simulink model "Modelos"  (R2025a)
settings: Solver=FixedStepDiscrete  StartTime=0.0  StopTime=P.Tsim  FixedStep=P.Ts  RelTol=1e-3
InitFcn:
  | CarregaDados
values from neighbouring files (symbols this model uses):
  P = struct    [CarregaDados.m]
(part 1 of 2)
settings Model: Creator=leize  LastModifiedBy=Rafael

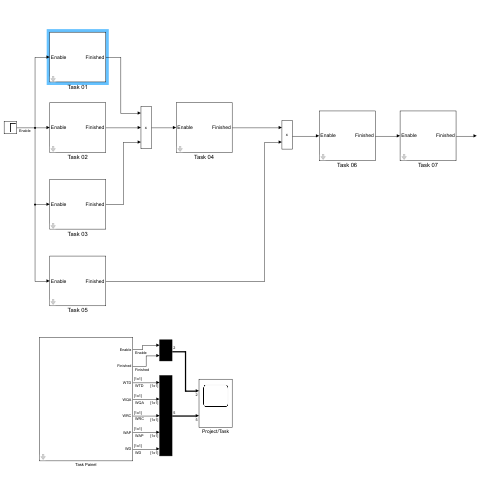
[thumbnail: Simulink's stored preview of the top-level diagram]
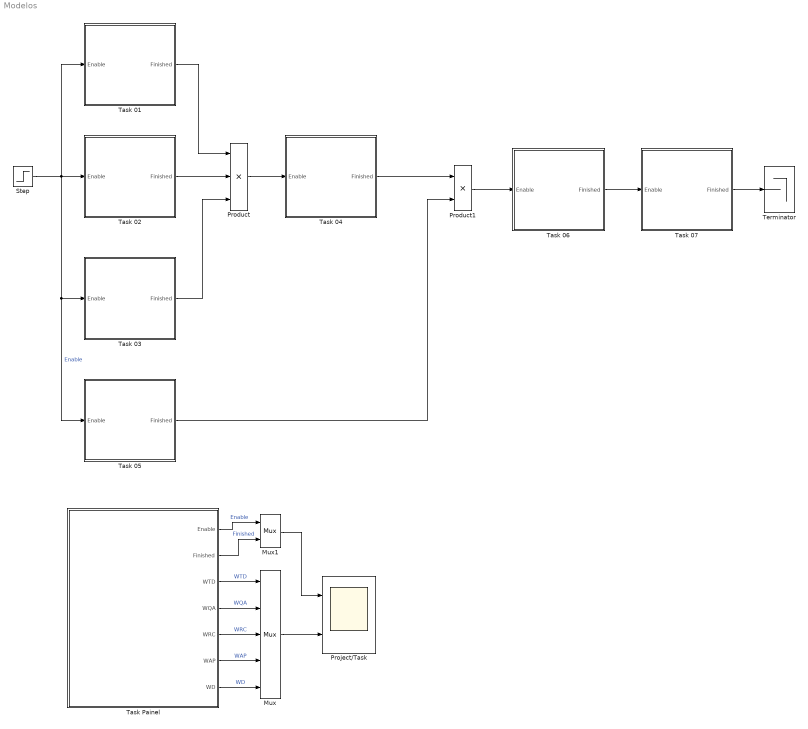
== system Modelos ==
  Mux : Mux  Inputs=5
  Mux1 : Mux  Inputs=2
  Product : Product  Inputs=3
  Product1 : Product
  Project/Task : Scope  NumInputPorts=2
      settings: ActiveDisplayYMinimum=-0.125  ActiveDisplayYMaximum=1.125  DataLoggingVariableName=ScopeData2
  Step : Step  Time=10  SampleTime=0
  Task 01 : Subsystem  mask{P=P, task_id=1}
      mask prompts: P "General task parameters"; task_id "Task Id (num)"
  Task 02 : Subsystem  mask{P=P, task_id=2}
      mask prompts: P "General task parameters"; task_id "Task Id (num)"
  Task 03 : Subsystem  mask{P=P, task_id=3}
      mask prompts: P "General task parameters"; task_id "Task Id (num)"
  Task 04 : Subsystem  mask{P=P, task_id=4}
      mask prompts: P "General task parameters"; task_id "Task Id (num)"
  Task 05 : Subsystem  mask{P=P, task_id=5}
      mask prompts: P "General task parameters"; task_id "Task Id (num)"
  Task 06 : Subsystem  mask{P=P, task_id=6}
      mask prompts: P "General task parameters"; task_id "Task Id (num)"
  Task 07 : Subsystem  mask{P=P, task_id=7}
      mask prompts: P "General task parameters"; task_id "Task Id (num)"
  Task Painel : Subsystem  mask{task_id=All Projet}
      mask prompts: task_id "Task Selecion"
  Terminator : Terminator
  wires:
  Task Painel/3(WTD) -> Mux/1  "WTD"
  Task Painel/6(WAP) -> Mux/4  "WAP"
  Task Painel/5(WRC) -> Mux/3  "WRC"
  Task Painel/4(WQA) -> Mux/2  "WQA"
  Task Painel/7(WD) -> Mux/5  "WD"
  Mux/1 -> Project/Task/2
  Step/1 -> Task 02/1(Enable), Task 01/1(Enable), Task 05/1(Enable), Task 03/1(Enable)  "Enable"
  Product/1 -> Task 04/1(Enable)
  Task 01/1(Finished) -> Product/1
  Task 02/1(Finished) -> Product/2
  Task 03/1(Finished) -> Product/3
  Task 04/1(Finished) -> Product1/1
  Task 05/1(Finished) -> Product1/2
  Product1/1 -> Task 06/1(Enable)
  Task 06/1(Finished) -> Task 07/1(Enable)
  Task 07/1(Finished) -> Terminator/1
  Mux1/1 -> Project/Task/1
  Task Painel/1(Enable) -> Mux1/1  "Enable"
  Task Painel/2(Finished) -> Mux1/2  "Finished"

== system Modelos/Task 01 ==
  Enable : Inport
  Controle : Subsystem
  Equações Modelo Discretizado : Subsystem
  MATLAB Function : MATLAB Function  TreatAsAtomicUnit=on
  Mux1 : Mux  Inputs=5
  Finished : Outport
  tag scope: Enable1=global, Finished1=global, W1=global
  wires:
  MATLAB Function/1(Done) -> Finished/1, [Finished1]  "Finished"
  Controle/1(Ações) -> Equações Modelo Discretizado/2(Ações)
  Enable/1 -> Equações Modelo Discretizado/1(Enable), MATLAB Function/1(enable), [Enable1]  "Enable"
  Equações Modelo Discretizado/3(Work Reviewing By Client) -> Mux1/3  "WRC"
  Equações Modelo Discretizado/1(Work To Do) -> Mux1/1  "WTD"
  Mux1/1 -> Controle/1(Estados Atuais), MATLAB Function/2(Work), [W1]
  Equações Modelo Discretizado/5(Work Done) -> Mux1/5  "WD"
  Equações Modelo Discretizado/4(Work Approved) -> Mux1/4  "WAP"
  Equações Modelo Discretizado/2("Work Awaiting quality assessment ") -> Mux1/2  "WQA"

== system Modelos/Task 02 ==
  Enable : Inport
  Controle : Subsystem
  Equações Modelo Discretizado : Subsystem
  MATLAB Function : MATLAB Function  TreatAsAtomicUnit=on
  Mux1 : Mux  Inputs=5
  Finished : Outport
  tag scope: Enable2=global, Finished2=global, W2=global
  wires:
  Equações Modelo Discretizado/2("Work Awaiting quality assessment ") -> Mux1/2  "WQA"
  Equações Modelo Discretizado/4(Work Approved) -> Mux1/4  "WAP"
  Equações Modelo Discretizado/5(Work Done) -> Mux1/5  "WD"
  Mux1/1 -> [W2], MATLAB Function/2(Work), Controle/1(Estados Atuais)
  Equações Modelo Discretizado/1(Work To Do) -> Mux1/1  "WTD"
  Equações Modelo Discretizado/3(Work Reviewing By Client) -> Mux1/3  "WRC"
  Enable/1 -> [Enable2], MATLAB Function/1(enable), Equações Modelo Discretizado/1(Enable)  "Enable"
  Controle/1(Ações) -> Equações Modelo Discretizado/2(Ações)
  MATLAB Function/1(Done) -> [Finished2], Finished/1  "Finished"

== system Modelos/Task 03 ==
  Enable : Inport
  Controle : Subsystem
  Equações Modelo Discretizado : Subsystem
  MATLAB Function : MATLAB Function  TreatAsAtomicUnit=on
  Mux1 : Mux  Inputs=5
  Finished : Outport
  tag scope: Enable3=global, Finished3=global, W3=global
  wires:
  MATLAB Function/1(Done) -> Finished/1, [Finished3]  "Finished"
  Controle/1(Ações) -> Equações Modelo Discretizado/2(Ações)
  Enable/1 -> Equações Modelo Discretizado/1(Enable), MATLAB Function/1(enable), [Enable3]  "Enable"
  Equações Modelo Discretizado/3(Work Reviewing By Client) -> Mux1/3  "WRC"
  Equações Modelo Discretizado/1(Work To Do) -> Mux1/1  "WTD"
  Mux1/1 -> Controle/1(Estados Atuais), MATLAB Function/2(Work), [W3]
  Equações Modelo Discretizado/5(Work Done) -> Mux1/5  "WD"
  Equações Modelo Discretizado/4(Work Approved) -> Mux1/4  "WAP"
  Equações Modelo Discretizado/2("Work Awaiting quality assessment ") -> Mux1/2  "WQA"

== system Modelos/Task 04 ==
  Enable : Inport
  Controle : Subsystem
  Equações Modelo Discretizado : Subsystem
  MATLAB Function : MATLAB Function  TreatAsAtomicUnit=on
  Mux1 : Mux  Inputs=5
  Finished : Outport
  tag scope: Enable4=global, Finished4=global, W4=global
  wires:
  Equações Modelo Discretizado/2("Work Awaiting quality assessment ") -> Mux1/2  "WQA"
  Equações Modelo Discretizado/4(Work Approved) -> Mux1/4  "WAP"
  Equações Modelo Discretizado/5(Work Done) -> Mux1/5  "WD"
  Mux1/1 -> [W4], MATLAB Function/2(Work), Controle/1(Estados Atuais)
  Equações Modelo Discretizado/1(Work To Do) -> Mux1/1  "WTD"
  Equações Modelo Discretizado/3(Work Reviewing By Client) -> Mux1/3  "WRC"
  Enable/1 -> [Enable4], MATLAB Function/1(enable), Equações Modelo Discretizado/1(Enable)  "Enable"
  Controle/1(Ações) -> Equações Modelo Discretizado/2(Ações)
  MATLAB Function/1(Done) -> [Finished4], Finished/1  "Finished"

== system Modelos/Task 05 ==
  Enable : Inport
  Controle : Subsystem
  Equações Modelo Discretizado : Subsystem
  MATLAB Function : MATLAB Function  TreatAsAtomicUnit=on
  Mux1 : Mux  Inputs=5
  Finished : Outport
  tag scope: Enable5=global, Finished5=global, W5=global
  wires:
  MATLAB Function/1(Done) -> Finished/1, [Finished5]  "Finished"
  Controle/1(Ações) -> Equações Modelo Discretizado/2(Ações)
  Enable/1 -> Equações Modelo Discretizado/1(Enable), MATLAB Function/1(enable), [Enable5]  "Enable"
  Equações Modelo Discretizado/3(Work Reviewing By Client) -> Mux1/3  "WRC"
  Equações Modelo Discretizado/1(Work To Do) -> Mux1/1  "WTD"
  Mux1/1 -> Controle/1(Estados Atuais), MATLAB Function/2(Work), [W5]
  Equações Modelo Discretizado/5(Work Done) -> Mux1/5  "WD"
  Equações Modelo Discretizado/4(Work Approved) -> Mux1/4  "WAP"
  Equações Modelo Discretizado/2("Work Awaiting quality assessment ") -> Mux1/2  "WQA"

== system Modelos/Task 06 ==
  Enable : Inport
  Controle : Subsystem
  Equações Modelo Discretizado : Subsystem
  MATLAB Function : MATLAB Function  TreatAsAtomicUnit=on
  Mux1 : Mux  Inputs=5
  Finished : Outport
  tag scope: Enable6=global, Finished6=global, W6=global
  wires:
  MATLAB Function/1(Done) -> Finished/1, [Finished6]  "Finished"
  Controle/1(Ações) -> Equações Modelo Discretizado/2(Ações)
  Enable/1 -> Equações Modelo Discretizado/1(Enable), MATLAB Function/1(enable), [Enable6]  "Enable"
  Equações Modelo Discretizado/3(Work Reviewing By Client) -> Mux1/3  "WRC"
  Equações Modelo Discretizado/1(Work To Do) -> Mux1/1  "WTD"
  Mux1/1 -> Controle/1(Estados Atuais), MATLAB Function/2(Work), [W6]
  Equações Modelo Discretizado/5(Work Done) -> Mux1/5  "WD"
  Equações Modelo Discretizado/4(Work Approved) -> Mux1/4  "WAP"
  Equações Modelo Discretizado/2("Work Awaiting quality assessment ") -> Mux1/2  "WQA"

== system Modelos/Task 07 ==
  Enable : Inport
  Controle : Subsystem
  Equações Modelo Discretizado : Subsystem
  MATLAB Function : MATLAB Function  TreatAsAtomicUnit=on
  Mux1 : Mux  Inputs=5
  Finished : Outport
  tag scope: Enable7=global, Finished7=global, W7=global
  wires:
  Equações Modelo Discretizado/2("Work Awaiting quality assessment ") -> Mux1/2  "WQA"
  Equações Modelo Discretizado/4(Work Approved) -> Mux1/4  "WAP"
  Equações Modelo Discretizado/5(Work Done) -> Mux1/5  "WD"
  Mux1/1 -> [W7], MATLAB Function/2(Work), Controle/1(Estados Atuais)
  Equações Modelo Discretizado/1(Work To Do) -> Mux1/1  "WTD"
  Equações Modelo Discretizado/3(Work Reviewing By Client) -> Mux1/3  "WRC"
  Enable/1 -> [Enable7], MATLAB Function/1(enable), Equações Modelo Discretizado/1(Enable)  "Enable"
  Controle/1(Ações) -> Equações Modelo Discretizado/2(Ações)
  MATLAB Function/1(Done) -> [Finished7], Finished/1  "Finished"

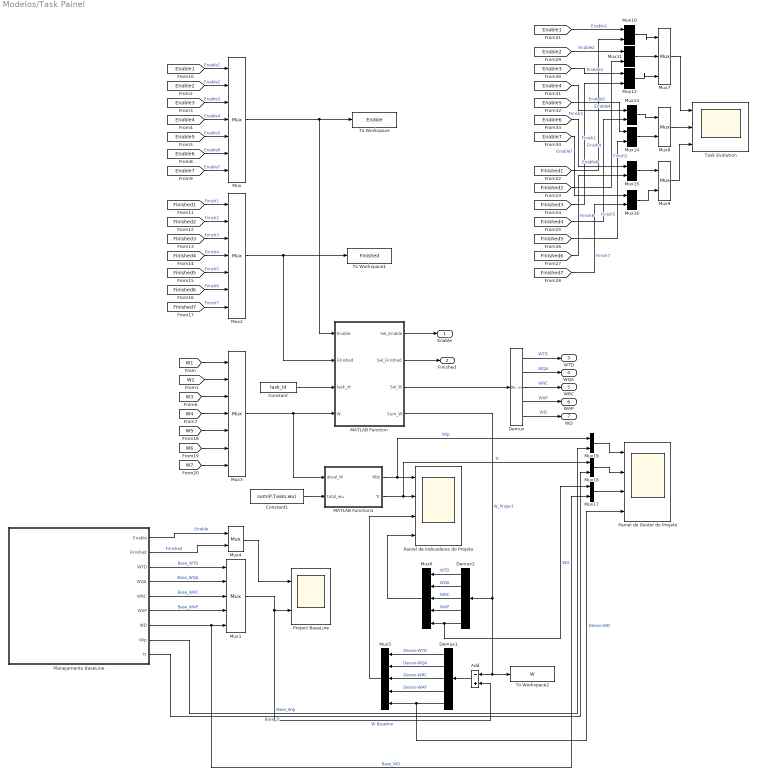
== system Modelos/Task Painel ==
  Add : Sum  Inputs=-+
  Constant : Constant  Value=task_id
  Constant1 : Constant  Value=sum(P.Tasks.wu)
  Demux : Demux  Outputs=5
  Demux1 : Demux  Outputs=5
  Demux2 : Demux  Outputs=5
  MATLAB Function : MATLAB Function  TreatAsAtomicUnit=on
  MATLAB Function1 : MATLAB Function  TreatAsAtomicUnit=on
  Mux : Mux  Inputs=7
  Mux1 : Mux  Inputs=5
  Mux{4,8..19} (13 alike) : Mux  Inputs=2
  Mux2 : Mux  Inputs=7
  Mux3 : Mux  Inputs=7
  Mux5 : Mux  Inputs=5
  Mux6 : Mux  Inputs=5
  Mux7 : Mux  Inputs=3
  Painel de Indicadores do Projeto : Scope  NumInputPorts=4
      settings: ActiveDisplayYMinimum=-25806.89231  ActiveDisplayYMaximum=232262.03078
  Painel do Gestor do Projeto : Scope  NumInputPorts=4
      settings: ActiveDisplayYMinimum=-25804.64462  ActiveDisplayYMaximum=232241.80155  DataLoggingVariableName=ScopeData2
  Planejamento BaseLine : Subsystem
  Project BaseLine : Scope  NumInputPorts=2
      settings: ActiveDisplayYMinimum=-0.125  ActiveDisplayYMaximum=1.125  DataLoggingVariableName=ScopeData2
  Task Evolution : Scope  NumInputPorts=3
      settings: ActiveDisplayYMinimum=-0.125  ActiveDisplayYMaximum=1.125
  To Workspace : ToWorkspace  VariableName=Enable  SampleTime=P.Ts
      settings: Save2DSignal=2-D array (concatenate along first dimension)
  To Workspace1 : ToWorkspace  VariableName=Finished  SampleTime=P.Ts
      settings: Save2DSignal=2-D array (concatenate along first dimension)
  To Workspace2 : ToWorkspace  VariableName=W  SampleTime=P.Ts
      settings: Save2DSignal=2-D array (concatenate along first dimension)
  Enable : Outport
  Finished : Outport  Port=2
  WTD : Outport  Port=3
  WQA : Outport  Port=4
  WRC : Outport  Port=5
  WAP : Outport  Port=6
  WD : Outport  Port=7
  wires:
  [W1] -> Mux3/1
  [W2] -> Mux3/2
  Demux/1 -> WTD/1  "WTD"
  Demux/2 -> WQA/1  "WQA"
  Demux/3 -> WRC/1  "WRC"
  Demux/4 -> WAP/1  "WAP"
  Demux/5 -> WD/1  "WD"
  Constant/1 -> MATLAB Function/3(task_id)
  [Enable2] -> Mux/2  "Enable2"
  [Enable3] -> Mux/3  "Enable3"
  Mux/1 -> To Workspace/1, MATLAB Function/1(Enable)
  [Enable4] -> Mux/4  "Enable4"
  [Enable5] -> Mux/5  "Enable5"
  [W3] -> Mux3/3
  [W4] -> Mux3/4
  [Enable6] -> Mux/6  "Enable6"
  [Enable7] -> Mux/7  "Enable7"
  [Enable1] -> Mux/1  "Enable1"
  [Finished1] -> Mux2/1  "Finish1"
  [Finished7] -> Mux2/7  "Finish7"
  [Finished6] -> Mux2/6  "Finish6"
  [Finished5] -> Mux2/5  "Finish5"
  [Finished4] -> Mux2/4  "Finish4"
  Mux2/1 -> To Workspace1/1, MATLAB Function/2(Finished)
  [Finished3] -> Mux2/3  "Finish3"
  [Finished2] -> Mux2/2  "Finish2"
  [W5] -> Mux3/5
  [W6] -> Mux3/6
  [W7] -> Mux3/7
  Mux3/1 -> MATLAB Function1/1(atual_W), MATLAB Function/4(W)
  MATLAB Function/1(Sel_Enable) -> Enable/1
  MATLAB Function/2(Sel_Finished) -> Finished/1
  Constant1/1 -> MATLAB Function1/2(total_wu)
  MATLAB Function1/1(Wip) -> Mux19/1, Painel de Indicadores do Projeto/1  "Wip"
  MATLAB Function1/2(Tr) -> Mux18/1, Painel de Indicadores do Projeto/2  "Tr"
  Planejamento BaseLine/1(Enable) -> Mux4/1  "Enable"
  Planejamento BaseLine/5(WRC) -> Mux1/3  "Base_WRC"
  Planejamento BaseLine/6(WAP) -> Mux1/4  "Base_WAP"
  Planejamento BaseLine/7(WD) -> Mux17/2, Mux1/5  "Base_WD"
  Planejamento BaseLine/3(WTD) -> Mux1/1  "Base_WTD"
  Mux4/1 -> Project BaseLine/1
  Mux1/1 -> Add/2, Project BaseLine/2  "W Baseline"
  Planejamento BaseLine/4(WQA) -> Mux1/2  "Base_WQA"
  MATLAB Function/3(Sel_W) -> Demux/1
  Planejamento BaseLine/2(Finished) -> Mux4/2  "Finished"
  MATLAB Function/4(Sum_W) -> Demux2/1, To Workspace2/1, Add/1  "W_Project"
  Add/1 -> Demux1/1
  Demux1/1 -> Mux5/1  "Desvio-WTD"
  Demux1/2 -> Mux5/2  "Desvio-WQA"
  Demux1/3 -> Mux5/3  "Desvio-WRC"
  Demux1/4 -> Mux5/4  "Desvio-WAP"
  Demux1/5 -> Painel do Gestor do Projeto/4, Mux5/5  "Desvio-WD"
  Mux5/1 -> Painel de Indicadores do Projeto/3
  Mux6/1 -> Painel de Indicadores do Projeto/4
  Demux2/5 -> Mux17/1, Mux6/5  "WD"
  Demux2/4 -> Mux6/4  "WAP"
  Demux2/3 -> Mux6/3  "WRC"
  Demux2/2 -> Mux6/2  "WQA"
  Demux2/1 -> Mux6/1  "WTD"
  [Enable4] -> Mux13/1  "Enable4"
  [Finished7] -> Mux16/2  "Finish7"
  [Enable3] -> Mux12/1  "Enable3"
  [Enable5] -> Mux14/1  "Enable5"
  [Finished1] -> Mux10/2  "Finish1"
  [Finished3] -> Mux12/2  "Finish3"
  [Finished5] -> Mux14/2  "Finish5"
  [Enable1] -> Mux10/1  "Enable1"
  [Finished4] -> Mux13/2  "Finish4"
  [Finished2] -> Mux11/2  "Finish2"
  [Finished6] -> Mux15/2  "Finish6"
  [Enable2] -> Mux11/1  "Enable2"
  [Enable6] -> Mux15/1  "Enable6"
  [Enable7] -> Mux16/1  "Enable7"
  Mux12/1 -> Mux7/3
  Mux11/1 -> Mux7/2
  Mux10/1 -> Mux7/1
  Mux7/1 -> Task Evolution/1
  Mux8/1 -> Task Evolution/2
  Mux9/1 -> Task Evolution/3
  Mux13/1 -> Mux8/1
  Mux14/1 -> Mux8/2
  Mux15/1 -> Mux9/1
  Mux16/1 -> Mux9/2
  Mux17/1 -> Painel do Gestor do Projeto/3
  Mux18/1 -> Painel do Gestor do Projeto/2
  Mux19/1 -> Painel do Gestor do Projeto/1
  Planejamento BaseLine/8(Wip) -> Mux19/2  "Base_Wip"
  Planejamento BaseLine/9(Tr) -> Mux18/2  "Base_Tr"

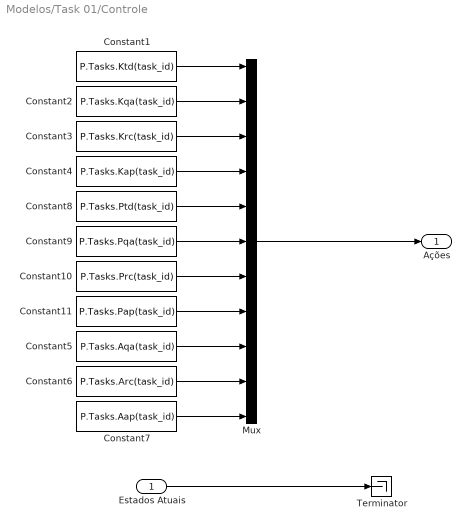
== system Modelos/Task 01/Controle ==
  Estados Atuais : Inport
  Constant1 : Constant  Value=P.Tasks.Ktd(task_id)
  Constant10 : Constant  Value=P.Tasks.Prc(task_id)
  Constant11 : Constant  Value=P.Tasks.Pap(task_id)
  Constant2 : Constant  Value=P.Tasks.Kqa(task_id)
  Constant3 : Constant  Value=P.Tasks.Krc(task_id)
  Constant4 : Constant  Value=P.Tasks.Kap(task_id)
  Constant5 : Constant  Value=P.Tasks.Aqa(task_id)
  Constant6 : Constant  Value=P.Tasks.Arc(task_id)
  Constant7 : Constant  Value=P.Tasks.Aap(task_id)
  Constant8 : Constant  Value=P.Tasks.Ptd(task_id)
  Constant9 : Constant  Value=P.Tasks.Pqa(task_id)
  Mux : Mux  Inputs=11
  Terminator : Terminator
  Ações : Outport
  wires:
  Estados Atuais/1 -> Terminator/1
  Constant1/1 -> Mux/1
  Constant4/1 -> Mux/4
  Constant3/1 -> Mux/3
  Constant2/1 -> Mux/2
  Mux/1 -> Ações/1
  Constant5/1 -> Mux/9
  Constant6/1 -> Mux/10
  Constant7/1 -> Mux/11
  Constant10/1 -> Mux/7
  Constant11/1 -> Mux/8
  Constant9/1 -> Mux/6
  Constant8/1 -> Mux/5

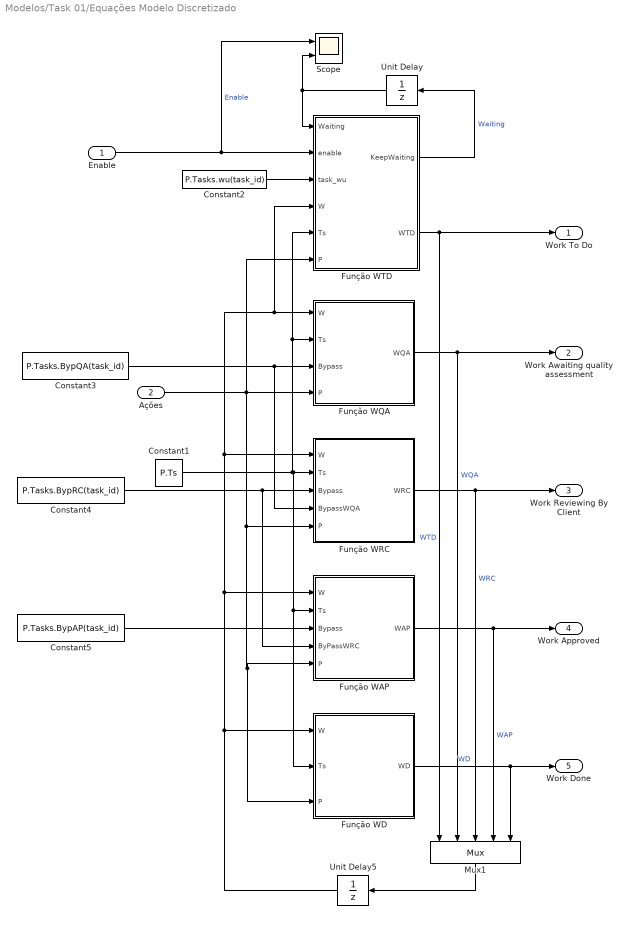
== system Modelos/Task 01/Equações Modelo Discretizado ==
  Enable : Inport
  Ações : Inport  Port=2
  Constant1 : Constant  Value=P.Ts  SampleTime=1
  Constant2 : Constant  Value=P.Tasks.wu(task_id)
  Constant3 : Constant  Value=P.Tasks.BypQA(task_id)  SampleTime=1
  Constant4 : Constant  Value=P.Tasks.BypRC(task_id)  SampleTime=1
  Constant5 : Constant  Value=P.Tasks.BypAP(task_id)  SampleTime=1
  Função WAP : MATLAB Function  TreatAsAtomicUnit=on
  Função WD : MATLAB Function  TreatAsAtomicUnit=on
  Função WQA : MATLAB Function  TreatAsAtomicUnit=on
  Função WRC : MATLAB Function  TreatAsAtomicUnit=on
  Função WTD : MATLAB Function  TreatAsAtomicUnit=on
  Mux1 : Mux  Inputs=5
  Scope : Scope  NumInputPorts=2
      settings: ActiveDisplayYMinimum=-0.125  ActiveDisplayYMaximum=1.125  DataLoggingVariableName=ScopeData2
  Unit Delay : UnitDelay  InitialCondition=1  SampleTime=-1  HasFrameUpgradeWarning=on
  Unit Delay5 : UnitDelay  InitialCondition=[P.Tasks.WTDini(task_id); P.Tasks.WQAini(task_id); P.Tasks.WRCini(task_id); P.Tasks.WAPini(task_id); P.Tasks.WDini(task_id)]  SampleTime=-1  HasFrameUpgradeWarning=on
  Work To Do : Outport
  "Work Awaiting quality assessment " : Outport  Port=2
  Work Reviewing By Client : Outport  Port=3
  Work Approved : Outport  Port=4
  Work Done : Outport  Port=5
  wires:
  Constant2/1 -> Função WTD/3(task_wu)
  Unit Delay/1 -> Scope/2, Função WTD/1(Waiting)
  Função WTD/1(KeepWaiting) -> Unit Delay/1  "Waiting"
  Função WD/1(WD) -> Mux1/5, Work Done/1  "WD"
  Constant1/1 -> Função WD/2(Ts), Função WAP/2(Ts), Função WRC/2(Ts), Função WQA/2(Ts), Função WTD/5(Ts)
  Unit Delay5/1 -> Função WD/1(W), Função WQA/1(W), Função WTD/4(W), Função WRC/1(W), Função WAP/1(W)
  Ações/1 -> Função WTD/6(P), Função WAP/5(P), Função WD/3(P), Função WRC/5(P), Função WQA/4(P)
  Mux1/1 -> Unit Delay5/1
  Enable/1 -> Função WTD/2(enable), Scope/1  "Enable"
  Função WAP/1(WAP) -> Mux1/4, Work Approved/1  "WAP"
  Função WRC/1(WRC) -> Mux1/3, Work Reviewing By Client/1  "WRC"
  Função WTD/2(WTD) -> Mux1/1, Work To Do/1  "WTD"
  Função WQA/1(WQA) -> Mux1/2, "Work Awaiting quality assessment "/1  "WQA"
  Constant3/1 -> Função WRC/4(BypassWQA), Função WQA/3(Bypass)
  Constant4/1 -> Função WAP/4(ByPassWRC), Função WRC/3(Bypass)
  Constant5/1 -> Função WAP/3(Bypass)

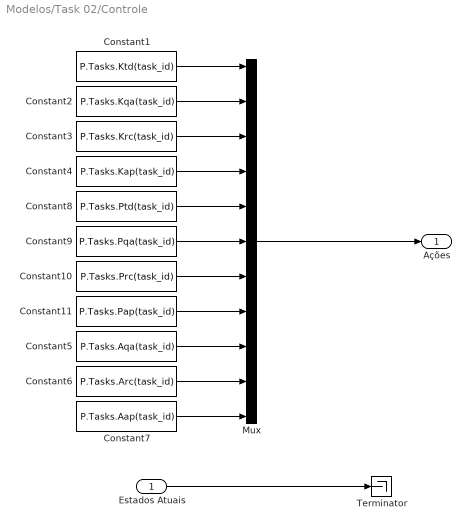
== system Modelos/Task 02/Controle ==
  Estados Atuais : Inport
  Constant1 : Constant  Value=P.Tasks.Ktd(task_id)
  Constant10 : Constant  Value=P.Tasks.Prc(task_id)
  Constant11 : Constant  Value=P.Tasks.Pap(task_id)
  Constant2 : Constant  Value=P.Tasks.Kqa(task_id)
  Constant3 : Constant  Value=P.Tasks.Krc(task_id)
  Constant4 : Constant  Value=P.Tasks.Kap(task_id)
  Constant5 : Constant  Value=P.Tasks.Aqa(task_id)
  Constant6 : Constant  Value=P.Tasks.Arc(task_id)
  Constant7 : Constant  Value=P.Tasks.Aap(task_id)
  Constant8 : Constant  Value=P.Tasks.Ptd(task_id)
  Constant9 : Constant  Value=P.Tasks.Pqa(task_id)
  Mux : Mux  Inputs=11
  Terminator : Terminator
  Ações : Outport
  wires:
  Constant8/1 -> Mux/5
  Constant9/1 -> Mux/6
  Constant11/1 -> Mux/8
  Constant10/1 -> Mux/7
  Constant7/1 -> Mux/11
  Constant6/1 -> Mux/10
  Constant5/1 -> Mux/9
  Mux/1 -> Ações/1
  Constant2/1 -> Mux/2
  Constant3/1 -> Mux/3
  Constant4/1 -> Mux/4
  Constant1/1 -> Mux/1
  Estados Atuais/1 -> Terminator/1

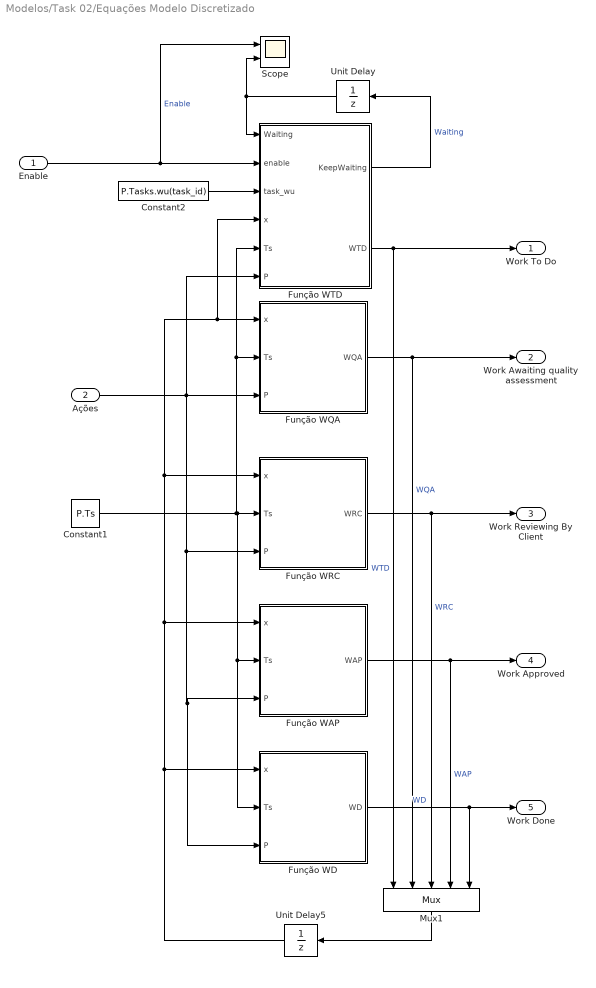
== system Modelos/Task 02/Equações Modelo Discretizado ==
  Enable : Inport
  Ações : Inport  Port=2
  Constant1 : Constant  Value=P.Ts  SampleTime=1
  Constant2 : Constant  Value=P.Tasks.wu(task_id)
  Função WAP : MATLAB Function  TreatAsAtomicUnit=on
  Função WD : MATLAB Function  TreatAsAtomicUnit=on
  Função WQA : MATLAB Function  TreatAsAtomicUnit=on
  Função WRC : MATLAB Function  TreatAsAtomicUnit=on
  Função WTD : MATLAB Function  TreatAsAtomicUnit=on
  Mux1 : Mux  Inputs=5
  Scope : Scope  NumInputPorts=2
      settings: ActiveDisplayYMinimum=-0.125  ActiveDisplayYMaximum=1.125  DataLoggingVariableName=ScopeData2
  Unit Delay : UnitDelay  InitialCondition=1  SampleTime=-1  HasFrameUpgradeWarning=on
  Unit Delay5 : UnitDelay  InitialCondition=[P.Tasks.WTDini(task_id); P.Tasks.WQAini(task_id); P.Tasks.WRCini(task_id); P.Tasks.WAPini(task_id); P.Tasks.WDini(task_id)]  SampleTime=-1  HasFrameUpgradeWarning=on
  Work To Do : Outport
  "Work Awaiting quality assessment " : Outport  Port=2
  Work Reviewing By Client : Outport  Port=3
  Work Approved : Outport  Port=4
  Work Done : Outport  Port=5
  wires:
  Função WQA/1(WQA) -> "Work Awaiting quality assessment "/1, Mux1/2  "WQA"
  Função WTD/2(WTD) -> Work To Do/1, Mux1/1  "WTD"
  Função WRC/1(WRC) -> Work Reviewing By Client/1, Mux1/3  "WRC"
  Função WAP/1(WAP) -> Work Approved/1, Mux1/4  "WAP"
  Enable/1 -> Scope/1, Função WTD/2(enable)  "Enable"
  Mux1/1 -> Unit Delay5/1
  Ações/1 -> Função WD/3(P), Função WAP/3(P), Função WRC/3(P), Função WTD/6(P), Função WQA/3(P)
  Unit Delay5/1 -> Função WRC/1(x), Função WTD/4(x), Função WQA/1(x), Função WAP/1(x), Função WD/1(x)
  Constant1/1 -> Função WRC/2(Ts), Função WD/2(Ts), Função WAP/2(Ts), Função WTD/5(Ts), Função WQA/2(Ts)
  Função WD/1(WD) -> Work Done/1, Mux1/5  "WD"
  Função WTD/1(KeepWaiting) -> Unit Delay/1  "Waiting"
  Unit Delay/1 -> Função WTD/1(Waiting), Scope/2
  Constant2/1 -> Função WTD/3(task_wu)

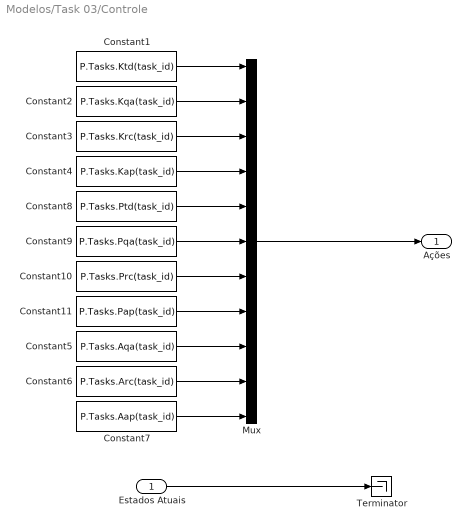
== system Modelos/Task 03/Controle ==
  Estados Atuais : Inport
  Constant1 : Constant  Value=P.Tasks.Ktd(task_id)
  Constant10 : Constant  Value=P.Tasks.Prc(task_id)
  Constant11 : Constant  Value=P.Tasks.Pap(task_id)
  Constant2 : Constant  Value=P.Tasks.Kqa(task_id)
  Constant3 : Constant  Value=P.Tasks.Krc(task_id)
  Constant4 : Constant  Value=P.Tasks.Kap(task_id)
  Constant5 : Constant  Value=P.Tasks.Aqa(task_id)
  Constant6 : Constant  Value=P.Tasks.Arc(task_id)
  Constant7 : Constant  Value=P.Tasks.Aap(task_id)
  Constant8 : Constant  Value=P.Tasks.Ptd(task_id)
  Constant9 : Constant  Value=P.Tasks.Pqa(task_id)
  Mux : Mux  Inputs=11
  Terminator : Terminator
  Ações : Outport
  wires:
  Estados Atuais/1 -> Terminator/1
  Constant1/1 -> Mux/1
  Constant4/1 -> Mux/4
  Constant3/1 -> Mux/3
  Constant2/1 -> Mux/2
  Mux/1 -> Ações/1
  Constant5/1 -> Mux/9
  Constant6/1 -> Mux/10
  Constant7/1 -> Mux/11
  Constant10/1 -> Mux/7
  Constant11/1 -> Mux/8
  Constant9/1 -> Mux/6
  Constant8/1 -> Mux/5

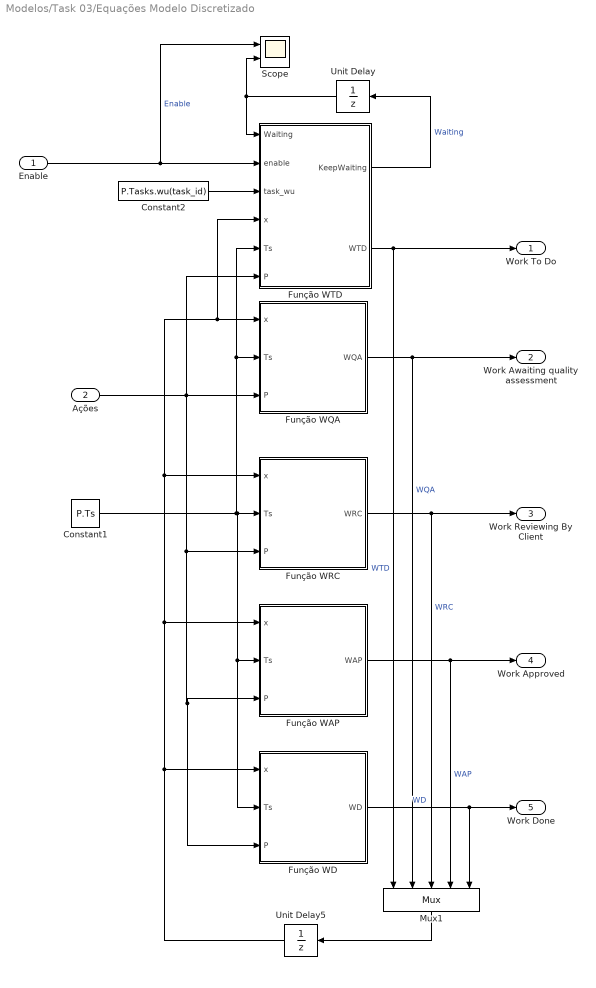
== system Modelos/Task 03/Equações Modelo Discretizado ==
  Enable : Inport
  Ações : Inport  Port=2
  Constant1 : Constant  Value=P.Ts  SampleTime=1
  Constant2 : Constant  Value=P.Tasks.wu(task_id)
  Função WAP : MATLAB Function  TreatAsAtomicUnit=on
  Função WD : MATLAB Function  TreatAsAtomicUnit=on
  Função WQA : MATLAB Function  TreatAsAtomicUnit=on
  Função WRC : MATLAB Function  TreatAsAtomicUnit=on
  Função WTD : MATLAB Function  TreatAsAtomicUnit=on
  Mux1 : Mux  Inputs=5
  Scope : Scope  NumInputPorts=2
      settings: ActiveDisplayYMinimum=-0.125  ActiveDisplayYMaximum=1.125  DataLoggingVariableName=ScopeData2
  Unit Delay : UnitDelay  InitialCondition=1  SampleTime=-1  HasFrameUpgradeWarning=on
  Unit Delay5 : UnitDelay  InitialCondition=[P.Tasks.WTDini(task_id); P.Tasks.WQAini(task_id); P.Tasks.WRCini(task_id); P.Tasks.WAPini(task_id); P.Tasks.WDini(task_id)]  SampleTime=-1  HasFrameUpgradeWarning=on
  Work To Do : Outport
  "Work Awaiting quality assessment " : Outport  Port=2
  Work Reviewing By Client : Outport  Port=3
  Work Approved : Outport  Port=4
  Work Done : Outport  Port=5
  wires:
  Constant2/1 -> Função WTD/3(task_wu)
  Unit Delay/1 -> Scope/2, Função WTD/1(Waiting)
  Função WTD/1(KeepWaiting) -> Unit Delay/1  "Waiting"
  Função WD/1(WD) -> Mux1/5, Work Done/1  "WD"
  Constant1/1 -> Função WQA/2(Ts), Função WTD/5(Ts), Função WAP/2(Ts), Função WD/2(Ts), Função WRC/2(Ts)
  Unit Delay5/1 -> Função WD/1(x), Função WAP/1(x), Função WQA/1(x), Função WTD/4(x), Função WRC/1(x)
  Ações/1 -> Função WQA/3(P), Função WTD/6(P), Função WRC/3(P), Função WAP/3(P), Função WD/3(P)
  Mux1/1 -> Unit Delay5/1
  Enable/1 -> Função WTD/2(enable), Scope/1  "Enable"
  Função WAP/1(WAP) -> Mux1/4, Work Approved/1  "WAP"
  Função WRC/1(WRC) -> Mux1/3, Work Reviewing By Client/1  "WRC"
  Função WTD/2(WTD) -> Mux1/1, Work To Do/1  "WTD"
  Função WQA/1(WQA) -> Mux1/2, "Work Awaiting quality assessment "/1  "WQA"

== system Modelos/Task 04/Controle ==
  Estados Atuais : Inport
  Constant1 : Constant  Value=P.Tasks.Ktd(task_id)
  Constant10 : Constant  Value=P.Tasks.Prc(task_id)
  Constant11 : Constant  Value=P.Tasks.Pap(task_id)
  Constant2 : Constant  Value=P.Tasks.Kqa(task_id)
  Constant3 : Constant  Value=P.Tasks.Krc(task_id)
  Constant4 : Constant  Value=P.Tasks.Kap(task_id)
  Constant5 : Constant  Value=P.Tasks.Aqa(task_id)
  Constant6 : Constant  Value=P.Tasks.Arc(task_id)
  Constant7 : Constant  Value=P.Tasks.Aap(task_id)
  Constant8 : Constant  Value=P.Tasks.Ptd(task_id)
  Constant9 : Constant  Value=P.Tasks.Pqa(task_id)
  Mux : Mux  Inputs=11
  Terminator : Terminator
  Ações : Outport
  wires:
  Constant8/1 -> Mux/5
  Constant9/1 -> Mux/6
  Constant11/1 -> Mux/8
  Constant10/1 -> Mux/7
  Constant7/1 -> Mux/11
  Constant6/1 -> Mux/10
  Constant5/1 -> Mux/9
  Mux/1 -> Ações/1
  Constant2/1 -> Mux/2
  Constant3/1 -> Mux/3
  Constant4/1 -> Mux/4
  Constant1/1 -> Mux/1
  Estados Atuais/1 -> Terminator/1

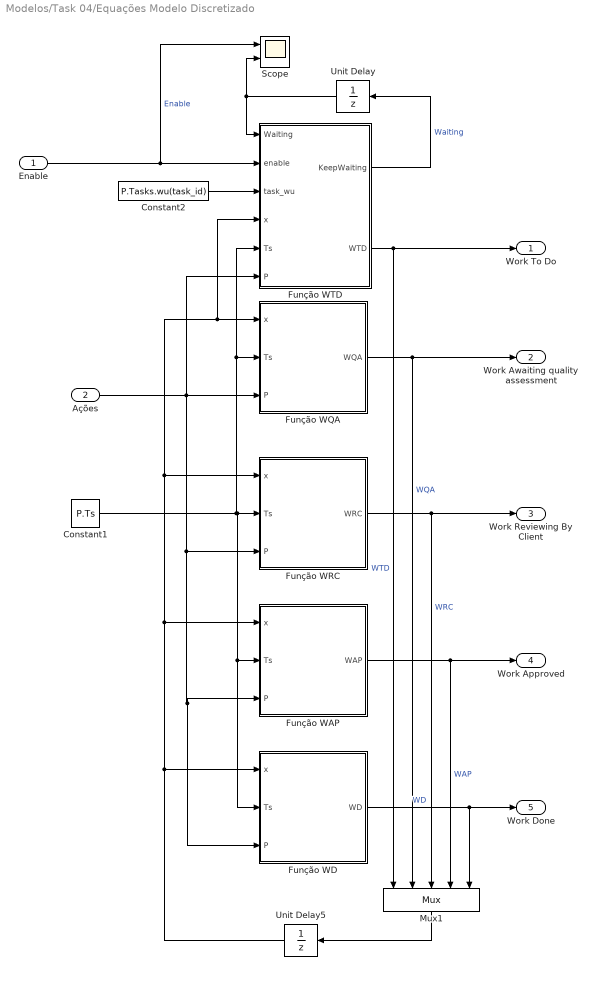
== system Modelos/Task 04/Equações Modelo Discretizado ==
  Enable : Inport
  Ações : Inport  Port=2
  Constant1 : Constant  Value=P.Ts  SampleTime=1
  Constant2 : Constant  Value=P.Tasks.wu(task_id)
  Função WAP : MATLAB Function  TreatAsAtomicUnit=on
  Função WD : MATLAB Function  TreatAsAtomicUnit=on
  Função WQA : MATLAB Function  TreatAsAtomicUnit=on
  Função WRC : MATLAB Function  TreatAsAtomicUnit=on
  Função WTD : MATLAB Function  TreatAsAtomicUnit=on
  Mux1 : Mux  Inputs=5
  Scope : Scope  NumInputPorts=2
      settings: ActiveDisplayYMinimum=-0.125  ActiveDisplayYMaximum=1.125  DataLoggingVariableName=ScopeData2
  Unit Delay : UnitDelay  InitialCondition=1  SampleTime=-1  HasFrameUpgradeWarning=on
  Unit Delay5 : UnitDelay  InitialCondition=[P.Tasks.WTDini(task_id); P.Tasks.WQAini(task_id); P.Tasks.WRCini(task_id); P.Tasks.WAPini(task_id); P.Tasks.WDini(task_id)]  SampleTime=-1  HasFrameUpgradeWarning=on
  Work To Do : Outport
  "Work Awaiting quality assessment " : Outport  Port=2
  Work Reviewing By Client : Outport  Port=3
  Work Approved : Outport  Port=4
  Work Done : Outport  Port=5
  wires:
  Função WQA/1(WQA) -> "Work Awaiting quality assessment "/1, Mux1/2  "WQA"
  Função WTD/2(WTD) -> Work To Do/1, Mux1/1  "WTD"
  Função WRC/1(WRC) -> Work Reviewing By Client/1, Mux1/3  "WRC"
  Função WAP/1(WAP) -> Work Approved/1, Mux1/4  "WAP"
  Enable/1 -> Scope/1, Função WTD/2(enable)  "Enable"
  Mux1/1 -> Unit Delay5/1
  Ações/1 -> Função WD/3(P), Função WAP/3(P), Função WRC/3(P), Função WTD/6(P), Função WQA/3(P)
  Unit Delay5/1 -> Função WRC/1(x), Função WTD/4(x), Função WQA/1(x), Função WAP/1(x), Função WD/1(x)
  Constant1/1 -> Função WRC/2(Ts), Função WD/2(Ts), Função WAP/2(Ts), Função WTD/5(Ts), Função WQA/2(Ts)
  Função WD/1(WD) -> Work Done/1, Mux1/5  "WD"
  Função WTD/1(KeepWaiting) -> Unit Delay/1  "Waiting"
  Unit Delay/1 -> Função WTD/1(Waiting), Scope/2
  Constant2/1 -> Função WTD/3(task_wu)

== system Modelos/Task 05/Controle ==
  Estados Atuais : Inport
  Constant1 : Constant  Value=P.Tasks.Ktd(task_id)
  Constant10 : Constant  Value=P.Tasks.Prc(task_id)
  Constant11 : Constant  Value=P.Tasks.Pap(task_id)
  Constant2 : Constant  Value=P.Tasks.Kqa(task_id)
  Constant3 : Constant  Value=P.Tasks.Krc(task_id)
  Constant4 : Constant  Value=P.Tasks.Kap(task_id)
  Constant5 : Constant  Value=P.Tasks.Aqa(task_id)
  Constant6 : Constant  Value=P.Tasks.Arc(task_id)
  Constant7 : Constant  Value=P.Tasks.Aap(task_id)
  Constant8 : Constant  Value=P.Tasks.Ptd(task_id)
  Constant9 : Constant  Value=P.Tasks.Pqa(task_id)
  Mux : Mux  Inputs=11
  Terminator : Terminator
  Ações : Outport
  wires:
  Estados Atuais/1 -> Terminator/1
  Constant1/1 -> Mux/1
  Constant4/1 -> Mux/4
  Constant3/1 -> Mux/3
  Constant2/1 -> Mux/2
  Mux/1 -> Ações/1
  Constant5/1 -> Mux/9
  Constant6/1 -> Mux/10
  Constant7/1 -> Mux/11
  Constant10/1 -> Mux/7
  Constant11/1 -> Mux/8
  Constant9/1 -> Mux/6
  Constant8/1 -> Mux/5

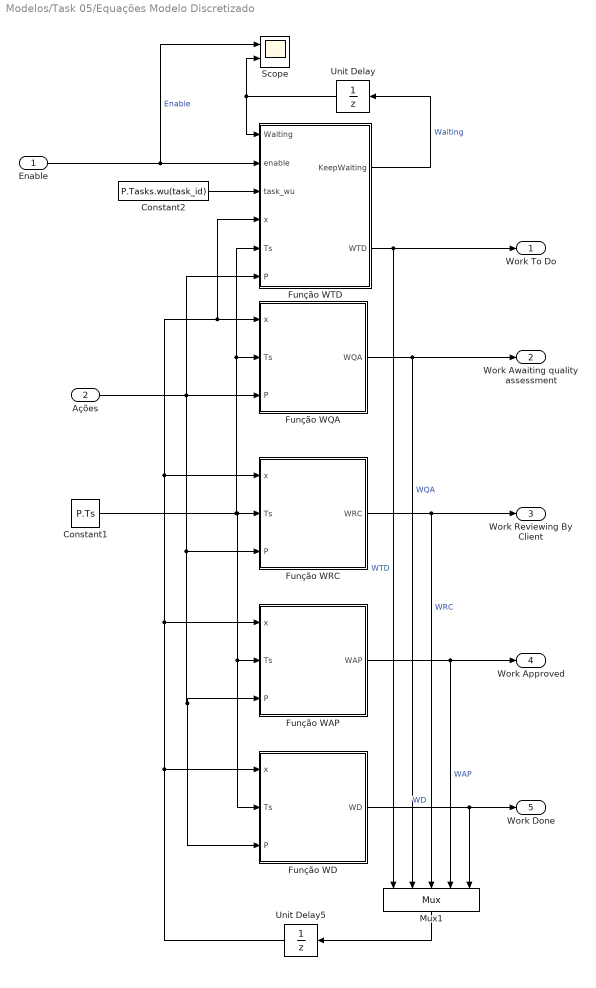
== system Modelos/Task 05/Equações Modelo Discretizado ==
  Enable : Inport
  Ações : Inport  Port=2
  Constant1 : Constant  Value=P.Ts  SampleTime=1
  Constant2 : Constant  Value=P.Tasks.wu(task_id)
  Função WAP : MATLAB Function  TreatAsAtomicUnit=on
  Função WD : MATLAB Function  TreatAsAtomicUnit=on
  Função WQA : MATLAB Function  TreatAsAtomicUnit=on
  Função WRC : MATLAB Function  TreatAsAtomicUnit=on
  Função WTD : MATLAB Function  TreatAsAtomicUnit=on
  Mux1 : Mux  Inputs=5
  Scope : Scope  NumInputPorts=2
      settings: ActiveDisplayYMinimum=-0.125  ActiveDisplayYMaximum=1.125  DataLoggingVariableName=ScopeData2
  Unit Delay : UnitDelay  InitialCondition=1  SampleTime=-1  HasFrameUpgradeWarning=on
  Unit Delay5 : UnitDelay  InitialCondition=[P.Tasks.WTDini(task_id); P.Tasks.WQAini(task_id); P.Tasks.WRCini(task_id); P.Tasks.WAPini(task_id); P.Tasks.WDini(task_id)]  SampleTime=-1  HasFrameUpgradeWarning=on
  Work To Do : Outport
  "Work Awaiting quality assessment " : Outport  Port=2
  Work Reviewing By Client : Outport  Port=3
  Work Approved : Outport  Port=4
  Work Done : Outport  Port=5
  wires:
  Constant2/1 -> Função WTD/3(task_wu)
  Unit Delay/1 -> Scope/2, Função WTD/1(Waiting)
  Função WTD/1(KeepWaiting) -> Unit Delay/1  "Waiting"
  Função WD/1(WD) -> Mux1/5, Work Done/1  "WD"
  Constant1/1 -> Função WQA/2(Ts), Função WTD/5(Ts), Função WAP/2(Ts), Função WD/2(Ts), Função WRC/2(Ts)
  Unit Delay5/1 -> Função WD/1(x), Função WAP/1(x), Função WQA/1(x), Função WTD/4(x), Função WRC/1(x)
  Ações/1 -> Função WQA/3(P), Função WTD/6(P), Função WRC/3(P), Função WAP/3(P), Função WD/3(P)
  Mux1/1 -> Unit Delay5/1
  Enable/1 -> Função WTD/2(enable), Scope/1  "Enable"
  Função WAP/1(WAP) -> Mux1/4, Work Approved/1  "WAP"
  Função WRC/1(WRC) -> Mux1/3, Work Reviewing By Client/1  "WRC"
  Função WTD/2(WTD) -> Mux1/1, Work To Do/1  "WTD"
  Função WQA/1(WQA) -> Mux1/2, "Work Awaiting quality assessment "/1  "WQA"

== system Modelos/Task 06/Controle ==
  Estados Atuais : Inport
  Constant1 : Constant  Value=P.Tasks.Ktd(task_id)
  Constant10 : Constant  Value=P.Tasks.Prc(task_id)
  Constant11 : Constant  Value=P.Tasks.Pap(task_id)
  Constant2 : Constant  Value=P.Tasks.Kqa(task_id)
  Constant3 : Constant  Value=P.Tasks.Krc(task_id)
  Constant4 : Constant  Value=P.Tasks.Kap(task_id)
  Constant5 : Constant  Value=P.Tasks.Aqa(task_id)
  Constant6 : Constant  Value=P.Tasks.Arc(task_id)
  Constant7 : Constant  Value=P.Tasks.Aap(task_id)
  Constant8 : Constant  Value=P.Tasks.Ptd(task_id)
  Constant9 : Constant  Value=P.Tasks.Pqa(task_id)
  Mux : Mux  Inputs=11
  Terminator : Terminator
  Ações : Outport
  wires:
  Estados Atuais/1 -> Terminator/1
  Constant1/1 -> Mux/1
  Constant4/1 -> Mux/4
  Constant3/1 -> Mux/3
  Constant2/1 -> Mux/2
  Mux/1 -> Ações/1
  Constant5/1 -> Mux/9
  Constant6/1 -> Mux/10
  Constant7/1 -> Mux/11
  Constant10/1 -> Mux/7
  Constant11/1 -> Mux/8
  Constant9/1 -> Mux/6
  Constant8/1 -> Mux/5

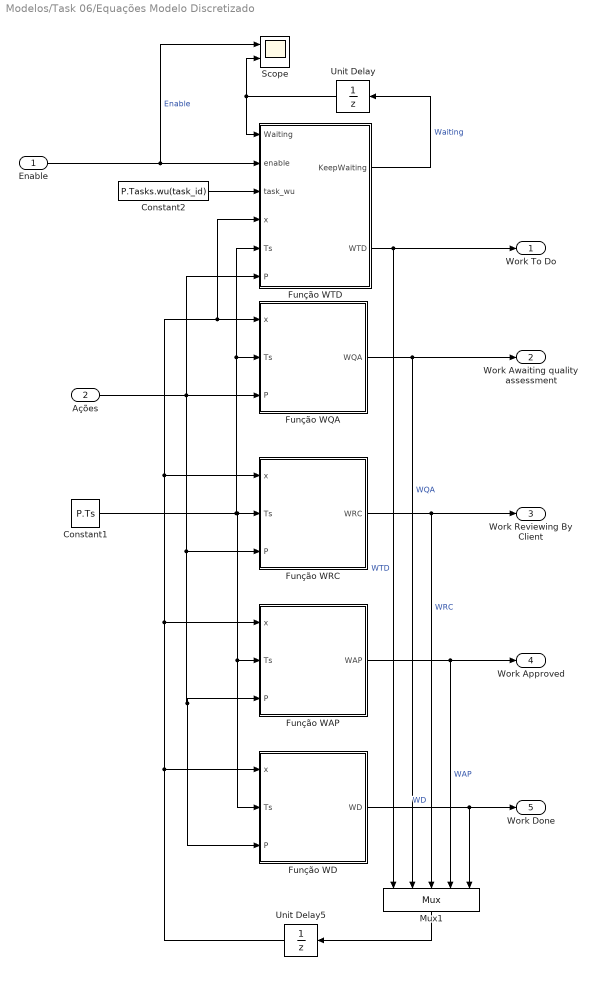
== system Modelos/Task 06/Equações Modelo Discretizado ==
  Enable : Inport
  Ações : Inport  Port=2
  Constant1 : Constant  Value=P.Ts  SampleTime=1
  Constant2 : Constant  Value=P.Tasks.wu(task_id)
  Função WAP : MATLAB Function  TreatAsAtomicUnit=on
  Função WD : MATLAB Function  TreatAsAtomicUnit=on
  Função WQA : MATLAB Function  TreatAsAtomicUnit=on
  Função WRC : MATLAB Function  TreatAsAtomicUnit=on
  Função WTD : MATLAB Function  TreatAsAtomicUnit=on
  Mux1 : Mux  Inputs=5
  Scope : Scope  NumInputPorts=2
      settings: ActiveDisplayYMinimum=-0.125  ActiveDisplayYMaximum=1.125  DataLoggingVariableName=ScopeData2
  Unit Delay : UnitDelay  InitialCondition=1  SampleTime=-1  HasFrameUpgradeWarning=on
  Unit Delay5 : UnitDelay  InitialCondition=[P.Tasks.WTDini(task_id); P.Tasks.WQAini(task_id); P.Tasks.WRCini(task_id); P.Tasks.WAPini(task_id); P.Tasks.WDini(task_id)]  SampleTime=-1  HasFrameUpgradeWarning=on
  Work To Do : Outport
  "Work Awaiting quality assessment " : Outport  Port=2
  Work Reviewing By Client : Outport  Port=3
  Work Approved : Outport  Port=4
  Work Done : Outport  Port=5
  wires:
  Constant2/1 -> Função WTD/3(task_wu)
  Unit Delay/1 -> Scope/2, Função WTD/1(Waiting)
  Função WTD/1(KeepWaiting) -> Unit Delay/1  "Waiting"
  Função WD/1(WD) -> Mux1/5, Work Done/1  "WD"
  Constant1/1 -> Função WQA/2(Ts), Função WTD/5(Ts), Função WAP/2(Ts), Função WD/2(Ts), Função WRC/2(Ts)
  Unit Delay5/1 -> Função WD/1(x), Função WAP/1(x), Função WQA/1(x), Função WTD/4(x), Função WRC/1(x)
  Ações/1 -> Função WQA/3(P), Função WTD/6(P), Função WRC/3(P), Função WAP/3(P), Função WD/3(P)
  Mux1/1 -> Unit Delay5/1
  Enable/1 -> Função WTD/2(enable), Scope/1  "Enable"
  Função WAP/1(WAP) -> Mux1/4, Work Approved/1  "WAP"
  Função WRC/1(WRC) -> Mux1/3, Work Reviewing By Client/1  "WRC"
  Função WTD/2(WTD) -> Mux1/1, Work To Do/1  "WTD"
  Função WQA/1(WQA) -> Mux1/2, "Work Awaiting quality assessment "/1  "WQA"

== system Modelos/Task 07/Controle ==
  Estados Atuais : Inport
  Constant1 : Constant  Value=P.Tasks.Ktd(task_id)
  Constant10 : Constant  Value=P.Tasks.Prc(task_id)
  Constant11 : Constant  Value=P.Tasks.Pap(task_id)
  Constant2 : Constant  Value=P.Tasks.Kqa(task_id)
  Constant3 : Constant  Value=P.Tasks.Krc(task_id)
  Constant4 : Constant  Value=P.Tasks.Kap(task_id)
  Constant5 : Constant  Value=P.Tasks.Aqa(task_id)
  Constant6 : Constant  Value=P.Tasks.Arc(task_id)
  Constant7 : Constant  Value=P.Tasks.Aap(task_id)
  Constant8 : Constant  Value=P.Tasks.Ptd(task_id)
  Constant9 : Constant  Value=P.Tasks.Pqa(task_id)
  Mux : Mux  Inputs=11
  Terminator : Terminator
  Ações : Outport
  wires:
  Constant8/1 -> Mux/5
  Constant9/1 -> Mux/6
  Constant11/1 -> Mux/8
  Constant10/1 -> Mux/7
  Constant7/1 -> Mux/11
  Constant6/1 -> Mux/10
  Constant5/1 -> Mux/9
  Mux/1 -> Ações/1
  Constant2/1 -> Mux/2
  Constant3/1 -> Mux/3
  Constant4/1 -> Mux/4
  Constant1/1 -> Mux/1
  Estados Atuais/1 -> Terminator/1

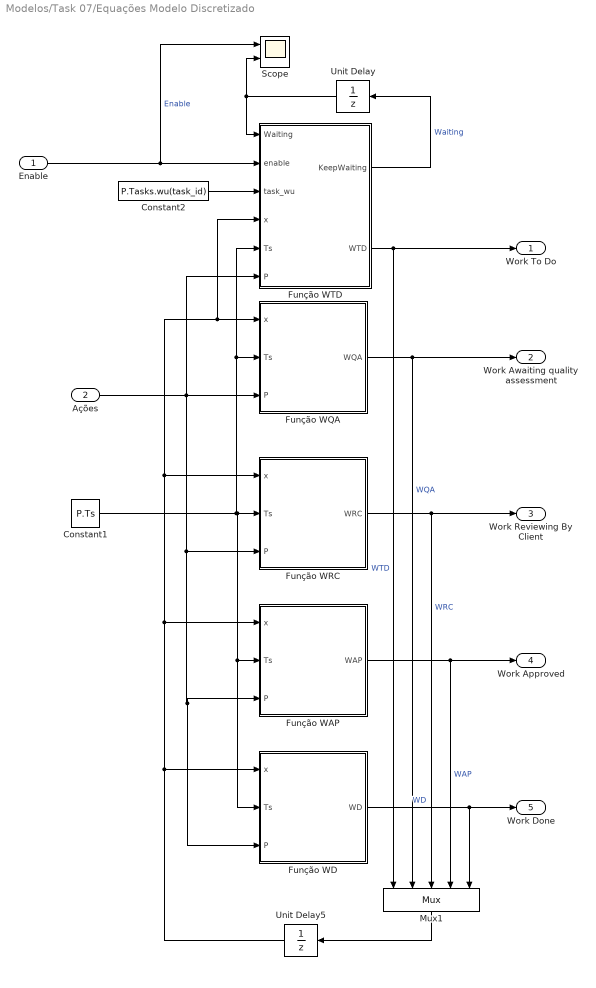
== system Modelos/Task 07/Equações Modelo Discretizado ==
  Enable : Inport
  Ações : Inport  Port=2
  Constant1 : Constant  Value=P.Ts  SampleTime=1
  Constant2 : Constant  Value=P.Tasks.wu(task_id)
  Função WAP : MATLAB Function  TreatAsAtomicUnit=on
  Função WD : MATLAB Function  TreatAsAtomicUnit=on
  Função WQA : MATLAB Function  TreatAsAtomicUnit=on
  Função WRC : MATLAB Function  TreatAsAtomicUnit=on
  Função WTD : MATLAB Function  TreatAsAtomicUnit=on
  Mux1 : Mux  Inputs=5
  Scope : Scope  NumInputPorts=2
      settings: ActiveDisplayYMinimum=-0.12499999999999997  ActiveDisplayYMaximum=1.125  DataLoggingVariableName=ScopeData2
  Unit Delay : UnitDelay  InitialCondition=1  SampleTime=-1  HasFrameUpgradeWarning=on
  Unit Delay5 : UnitDelay  InitialCondition=[P.Tasks.WTDini(task_id); P.Tasks.WQAini(task_id); P.Tasks.WRCini(task_id); P.Tasks.WAPini(task_id); P.Tasks.WDini(task_id)]  SampleTime=-1  HasFrameUpgradeWarning=on
  Work To Do : Outport
  "Work Awaiting quality assessment " : Outport  Port=2
  Work Reviewing By Client : Outport  Port=3
  Work Approved : Outport  Port=4
  Work Done : Outport  Port=5
  wires:
  Função WQA/1(WQA) -> "Work Awaiting quality assessment "/1, Mux1/2  "WQA"
  Função WTD/2(WTD) -> Work To Do/1, Mux1/1  "WTD"
  Função WRC/1(WRC) -> Work Reviewing By Client/1, Mux1/3  "WRC"
  Função WAP/1(WAP) -> Work Approved/1, Mux1/4  "WAP"
  Enable/1 -> Scope/1, Função WTD/2(enable)  "Enable"
  Mux1/1 -> Unit Delay5/1
  Ações/1 -> Função WD/3(P), Função WAP/3(P), Função WRC/3(P), Função WTD/6(P), Função WQA/3(P)
  Unit Delay5/1 -> Função WRC/1(x), Função WTD/4(x), Função WQA/1(x), Função WAP/1(x), Função WD/1(x)
  Constant1/1 -> Função WRC/2(Ts), Função WD/2(Ts), Função WAP/2(Ts), Função WTD/5(Ts), Função WQA/2(Ts)
  Função WD/1(WD) -> Work Done/1, Mux1/5  "WD"
  Função WTD/1(KeepWaiting) -> Unit Delay/1  "Waiting"
  Unit Delay/1 -> Função WTD/1(Waiting), Scope/2
  Constant2/1 -> Função WTD/3(task_wu)

== system Modelos/Task Painel/Planejamento BaseLine ==
  Add : Sum  Inputs=++++
  Constant1 : Constant  Value=sum(P.Tasks.wu)
  Demux : Demux  Outputs=7
  Divide : Product  Inputs=*/
  TabelaPlanejamento : FromWorkspace  VariableName=BaseLine  SampleTime=P.Ts  OutputAfterFinalValue=Holding final value
  Enable : Outport
  Finished : Outport  Port=2
  WTD : Outport  Port=3
  WQA : Outport  Port=4
  WRC : Outport  Port=5
  WAP : Outport  Port=6
  WD : Outport  Port=7
  Wip : Outport  Port=8
  Tr : Outport  Port=9
  wires:
  TabelaPlanejamento/1 -> Demux/1
  Demux/3 -> Add/1, WTD/1  "WTD"
  Demux/4 -> Add/2, WQA/1  "WQA"
  Demux/5 -> Add/3, WRC/1  "WRC"
  Demux/6 -> Add/4, WAP/1  "WAP"
  Demux/7 -> WD/1  "WD"
  Demux/1 -> Enable/1  "Enable"
  Demux/2 -> Finished/1  "Finished"
  Constant1/1 -> Divide/2
  Add/1 -> Divide/1, Wip/1
  Divide/1 -> Tr/1

== matlab function Modelos/Task 03/Equações Modelo Discretizado/Função WTD ==
  data: KeepWaiting output; Waiting input; enable input; task_wu input; x input; Ts input; WTD output; P input
function [KeepWaiting,WTD] = fcn(Waiting,enable,task_wu,x,Ts,P)
    % Estados atuais
    WTD=x(1);  WQA=x(2);
    WRC=x(3);  WAP=x(4);

    if Waiting & enable & sum(x)==0 % Valeu só para condição incial
        WTD=task_wu;    % Força condição inicial igual ao WU da respectiva atividade
        KeepWaiting=0;  % Não precisa mais esperar
    else
        KeepWaiting=1;  % Continuar esperando o ENABLE
    end

    % Extrai constantes dos parâmetros
    Ktd=P(1);     Kqa=P(2);      Krc=P(3);      Kap=P(4);
    Ptd=P(5);     Pqa=P(6);      Prc=P(7);      Pap=P(8);
    AlfaQA=P(9);  AlfaRC=P(10);  AlfaAP=P(11);
    
    % Calcula as entradas por retrabalho
    ReQA=AlfaQA*Kqa*sqrt(WQA+Pqa);  % Por revisão interna
    ReRC=AlfaRC*Krc*sqrt(WRC+Prc);  % Por solicitação do cliente
    ReAP=AlfaAP*Kap*sqrt(WAP+Pap);  % Por não aprovação final
    ReWork=ReQA+ReRC+ReAP;          % Total de retrabalho

    % Expressão da Eq.Diferencial
    Derivada = - Ktd*sqrt(WTD+Ptd) + ReWork;
    
    % Atualização do Estado
    WTD = WTD + Ts*Derivada;

    % Proteção, já que não faz sentido quantidades negativas para reciclos
    WTD=max(WTD,0);
end

== matlab function Modelos/Task 03/MATLAB Function ==
  data: enable input; Done output; Work input
function Done = fcn(enable,Work)
  
  if (enable) & (sum(Work(1:4))==0)   % Habilitado mas não tem mais nada para fazer
    Done = 1;  % Trabalho feito
  else
    Done = 0;  % Ainda há trabalho por fazer
  end
end

== matlab function Modelos/Task 04/Equações Modelo Discretizado/Função WAP ==
  data: x input; Ts input; WAP output; P input
function WAP = fcn(x,Ts,P)
    % Estados atuais
    WTD=x(1);  WQA=x(2);
    WRC=x(3);  WAP=x(4);

    % Extrai constantes dos parâmetros
    Ktd=P(1);     Kqa=P(2);      Krc=P(3);      Kap=P(4);
    Ptd=P(5);     Pqa=P(6);      Prc=P(7);      Pap=P(8);
    AlfaQA=P(9);  AlfaRC=P(10);  AlfaAP=P(11);

    % Entrada é a vazão de saida do tanque WRC, descontados os retrabalhos de RC
    Qin=(1-AlfaRC)*Krc*sqrt(WRC+Prc);  

    % Fluxo de saida de QAP
    Qout=Kap*sqrt(WAP+Pap);  % Saida para avaliar trabalho aprovado ou retrabalho por não aprovação

    % Expressão da Eq.Diferencial
    Derivada = Qin - Qout;
    
    % Atualização do Estado
    WAP = WAP + Ts*Derivada;

    % Proteção, já que não faz sentido quantidades negativas para reciclos
    WAP=max(WAP,0);
end

== matlab function Modelos/Task 04/Equações Modelo Discretizado/Função WD ==
  data: x input; Ts input; WD output; P input
function WD = fcn(x,Ts,P)
    % Estados atuais
    WTD=x(1);  WQA=x(2);
    WRC=x(3);  WAP=x(4);
    WD=x(5);

    % Extrai constantes dos parâmetros
    Ktd=P(1);     Kqa=P(2);      Krc=P(3);      Kap=P(4);
    Ptd=P(5);     Pqa=P(6);      Prc=P(7);      Pap=P(8);
    AlfaQA=P(9);  AlfaRC=P(10);  AlfaAP=P(11);

    % Entrada é a vazão de saida do tanque WAP, descontados os retrabalhos de AP
    Qin=(1-AlfaAP)*Kap*sqrt(WAP+Pap);  

    % Expressão da Eq.Diferencial
    Derivada = Qin;    % Só acumula infinitamente o trabalho realizado
    
    % Atualização do Estado
    WD = WD + Ts*Derivada;

    % Proteção, já que não faz sentido quantidades negativas para reciclos
    WD=max(WD,0);
end

== matlab function Modelos/Task 02/Equações Modelo Discretizado/Função WAP ==
  data: x input; Ts input; WAP output; P input
function WAP = fcn(x,Ts,P)
    % Estados atuais
    WTD=x(1);  WQA=x(2);
    WRC=x(3);  WAP=x(4);

    % Extrai constantes dos parâmetros
    Ktd=P(1);     Kqa=P(2);      Krc=P(3);      Kap=P(4);
    Ptd=P(5);     Pqa=P(6);      Prc=P(7);      Pap=P(8);
    AlfaQA=P(9);  AlfaRC=P(10);  AlfaAP=P(11);

    % Entrada é a vazão de saida do tanque WRC, descontados os retrabalhos de RC
    Qin=(1-AlfaRC)*Krc*sqrt(WRC+Prc);  

    % Fluxo de saida de QAP
    Qout=Kap*sqrt(WAP+Pap);  % Saida para avaliar trabalho aprovado ou retrabalho por não aprovação

    % Expressão da Eq.Diferencial
    Derivada = Qin - Qout;
    
    % Atualização do Estado
    WAP = WAP + Ts*Derivada;

    % Proteção, já que não faz sentido quantidades negativas para reciclos
    WAP=max(WAP,0);
end

== matlab function Modelos/Task 04/Equações Modelo Discretizado/Função WQA ==
  data: x input; Ts input; WQA output; P input
function WQA = fcn(x,Ts,P)
    % Estados atuais
    WTD=x(1);  WQA=x(2);
    WRC=x(3);  WAP=x(4);

    % Extrai constantes dos parâmetros
    Ktd=P(1);     Kqa=P(2);      Krc=P(3);      Kap=P(4);
    Ptd=P(5);     Pqa=P(6);      Prc=P(7);      Pap=P(8);
    AlfaQA=P(9);  AlfaRC=P(10);  AlfaAP=P(11);


    % Entrada é a vazão de saida do WTD
    Qin=Ktd*sqrt(WTD+Ptd);  

    % Fluxo de saida de QA
    Qout=Kqa*sqrt(WQA+Pqa);  % Saida para avaliar boa qualidade ou retrabalho

    % Expressão da Eq.Diferencial
    Derivada = Qin - Qout;
    
    % Atualização do Estado
    WQA = WQA + Ts*Derivada;

    % Proteção, já que não faz sentido quantidades negativas para reciclos
    WQA=max(WQA,0);
end

== matlab function Modelos/Task 04/Equações Modelo Discretizado/Função WRC ==
  data: x input; Ts input; WRC output; P input
function WRC = fcn(x,Ts,P)
    % Estados atuais
    WTD=x(1);  WQA=x(2);
    WRC=x(3);  WAP=x(4);

    % Extrai constantes dos parâmetros
    Ktd=P(1);     Kqa=P(2);      Krc=P(3);      Kap=P(4);
    Ptd=P(5);     Pqa=P(6);      Prc=P(7);      Pap=P(8);
    AlfaQA=P(9);  AlfaRC=P(10);  AlfaAP=P(11);

    % Entrada é a vazão de saida do tanque WQA, descontados os retrabalhos de QA
    Qin=(1-AlfaQA)*Kqa*sqrt(WQA+Pqa);  

    % Fluxo de saida de QRC
    Qout=Krc*sqrt(WRC+Prc);  % Saida para avaliar aprovação pelo cliente ou retrabalho

    % Expressão da Eq.Diferencial
    Derivada = Qin - Qout;
    
    % Atualização do Estado
    WRC = WRC + Ts*Derivada;

    % Proteção, já que não faz sentido quantidades negativas para reciclos
    WRC=max(WRC,0);
end

== matlab function Modelos/Task 04/Equações Modelo Discretizado/Função WTD ==
  data: KeepWaiting output; Waiting input; enable input; task_wu input; x input; Ts input; WTD output; P input
function [KeepWaiting,WTD] = fcn(Waiting,enable,task_wu,x,Ts,P)
    % Estados atuais
    WTD=x(1);  WQA=x(2);
    WRC=x(3);  WAP=x(4);

    if Waiting & enable & sum(x)==0 % Valeu só para condição incial
        WTD=task_wu;    % Força condição inicial igual ao WU da respectiva atividade
        KeepWaiting=0;  % Não precisa mais esperar
    else
        KeepWaiting=1;  % Continuar esperando o ENABLE
    end

    % Extrai constantes dos parâmetros
    Ktd=P(1);     Kqa=P(2);      Krc=P(3);      Kap=P(4);
    Ptd=P(5);     Pqa=P(6);      Prc=P(7);      Pap=P(8);
    AlfaQA=P(9);  AlfaRC=P(10);  AlfaAP=P(11);
    
    % Calcula as entradas por retrabalho
    ReQA=AlfaQA*Kqa*sqrt(WQA+Pqa);  % Por revisão interna
    ReRC=AlfaRC*Krc*sqrt(WRC+Prc);  % Por solicitação do cliente
    ReAP=AlfaAP*Kap*sqrt(WAP+Pap);  % Por não aprovação final
    ReWork=ReQA+ReRC+ReAP;          % Total de retrabalho

    % Expressão da Eq.Diferencial
    Derivada = - Ktd*sqrt(WTD+Ptd) + ReWork;
    
    % Atualização do Estado
    WTD = WTD + Ts*Derivada;

    % Proteção, já que não faz sentido quantidades negativas para reciclos
    WTD=max(WTD,0);
end

== matlab function Modelos/Task 04/MATLAB Function ==
  data: enable input; Done output; Work input
function Done = fcn(enable,Work)
  
  if (enable) & (sum(Work(1:4))==0)   % Habilitado mas não tem mais nada para fazer
    Done = 1;  % Trabalho feito
  else
    Done = 0;  % Ainda há trabalho por fazer
  end
end

== matlab function Modelos/Task 05/Equações Modelo Discretizado/Função WAP ==
  data: x input; Ts input; WAP output; P input
function WAP = fcn(x,Ts,P)
    % Estados atuais
    WTD=x(1);  WQA=x(2);
    WRC=x(3);  WAP=x(4);

    % Extrai constantes dos parâmetros
    Ktd=P(1);     Kqa=P(2);      Krc=P(3);      Kap=P(4);
    Ptd=P(5);     Pqa=P(6);      Prc=P(7);      Pap=P(8);
    AlfaQA=P(9);  AlfaRC=P(10);  AlfaAP=P(11);

    % Entrada é a vazão de saida do tanque WRC, descontados os retrabalhos de RC
    Qin=(1-AlfaRC)*Krc*sqrt(WRC+Prc);  

    % Fluxo de saida de QAP
    Qout=Kap*sqrt(WAP+Pap);  % Saida para avaliar trabalho aprovado ou retrabalho por não aprovação

    % Expressão da Eq.Diferencial
    Derivada = Qin - Qout;
    
    % Atualização do Estado
    WAP = WAP + Ts*Derivada;

    % Proteção, já que não faz sentido quantidades negativas para reciclos
    WAP=max(WAP,0);
end

== matlab function Modelos/Task 05/Equações Modelo Discretizado/Função WD ==
  data: x input; Ts input; WD output; P input
function WD = fcn(x,Ts,P)
    % Estados atuais
    WTD=x(1);  WQA=x(2);
    WRC=x(3);  WAP=x(4);
    WD=x(5);

    % Extrai constantes dos parâmetros
    Ktd=P(1);     Kqa=P(2);      Krc=P(3);      Kap=P(4);
    Ptd=P(5);     Pqa=P(6);      Prc=P(7);      Pap=P(8);
    AlfaQA=P(9);  AlfaRC=P(10);  AlfaAP=P(11);

    % Entrada é a vazão de saida do tanque WAP, descontados os retrabalhos de AP
    Qin=(1-AlfaAP)*Kap*sqrt(WAP+Pap);  

    % Expressão da Eq.Diferencial
    Derivada = Qin;    % Só acumula infinitamente o trabalho realizado
    
    % Atualização do Estado
    WD = WD + Ts*Derivada;

    % Proteção, já que não faz sentido quantidades negativas para reciclos
    WD=max(WD,0);
end

== matlab function Modelos/Task 05/Equações Modelo Discretizado/Função WQA ==
  data: x input; Ts input; WQA output; P input
function WQA = fcn(x,Ts,P)
    % Estados atuais
    WTD=x(1);  WQA=x(2);
    WRC=x(3);  WAP=x(4);

    % Extrai constantes dos parâmetros
    Ktd=P(1);     Kqa=P(2);      Krc=P(3);      Kap=P(4);
    Ptd=P(5);     Pqa=P(6);      Prc=P(7);      Pap=P(8);
    AlfaQA=P(9);  AlfaRC=P(10);  AlfaAP=P(11);


    % Entrada é a vazão de saida do WTD
    Qin=Ktd*sqrt(WTD+Ptd);  

    % Fluxo de saida de QA
    Qout=Kqa*sqrt(WQA+Pqa);  % Saida para avaliar boa qualidade ou retrabalho

    % Expressão da Eq.Diferencial
    Derivada = Qin - Qout;
    
    % Atualização do Estado
    WQA = WQA + Ts*Derivada;

    % Proteção, já que não faz sentido quantidades negativas para reciclos
    WQA=max(WQA,0);
end

== matlab function Modelos/Task 05/Equações Modelo Discretizado/Função WRC ==
  data: x input; Ts input; WRC output; P input
function WRC = fcn(x,Ts,P)
    % Estados atuais
    WTD=x(1);  WQA=x(2);
    WRC=x(3);  WAP=x(4);

    % Extrai constantes dos parâmetros
    Ktd=P(1);     Kqa=P(2);      Krc=P(3);      Kap=P(4);
    Ptd=P(5);     Pqa=P(6);      Prc=P(7);      Pap=P(8);
    AlfaQA=P(9);  AlfaRC=P(10);  AlfaAP=P(11);

    % Entrada é a vazão de saida do tanque WQA, descontados os retrabalhos de QA
    Qin=(1-AlfaQA)*Kqa*sqrt(WQA+Pqa);  

    % Fluxo de saida de QRC
    Qout=Krc*sqrt(WRC+Prc);  % Saida para avaliar aprovação pelo cliente ou retrabalho

    % Expressão da Eq.Diferencial
    Derivada = Qin - Qout;
    
    % Atualização do Estado
    WRC = WRC + Ts*Derivada;

    % Proteção, já que não faz sentido quantidades negativas para reciclos
    WRC=max(WRC,0);
end

== matlab function Modelos/Task 05/Equações Modelo Discretizado/Função WTD ==
  data: KeepWaiting output; Waiting input; enable input; task_wu input; x input; Ts input; WTD output; P input
function [KeepWaiting,WTD] = fcn(Waiting,enable,task_wu,x,Ts,P)
    % Estados atuais
    WTD=x(1);  WQA=x(2);
    WRC=x(3);  WAP=x(4);

    if Waiting & enable & sum(x)==0 % Valeu só para condição incial
        WTD=task_wu;    % Força condição inicial igual ao WU da respectiva atividade
        KeepWaiting=0;  % Não precisa mais esperar
    else
        KeepWaiting=1;  % Continuar esperando o ENABLE
    end

    % Extrai constantes dos parâmetros
    Ktd=P(1);     Kqa=P(2);      Krc=P(3);      Kap=P(4);
    Ptd=P(5);     Pqa=P(6);      Prc=P(7);      Pap=P(8);
    AlfaQA=P(9);  AlfaRC=P(10);  AlfaAP=P(11);
    
    % Calcula as entradas por retrabalho
    ReQA=AlfaQA*Kqa*sqrt(WQA+Pqa);  % Por revisão interna
    ReRC=AlfaRC*Krc*sqrt(WRC+Prc);  % Por solicitação do cliente
    ReAP=AlfaAP*Kap*sqrt(WAP+Pap);  % Por não aprovação final
    ReWork=ReQA+ReRC+ReAP;          % Total de retrabalho

    % Expressão da Eq.Diferencial
    Derivada = - Ktd*sqrt(WTD+Ptd) + ReWork;
    
    % Atualização do Estado
    WTD = WTD + Ts*Derivada;

    % Proteção, já que não faz sentido quantidades negativas para reciclos
    WTD=max(WTD,0);
end

== matlab function Modelos/Task 02/Equações Modelo Discretizado/Função WD ==
  data: x input; Ts input; WD output; P input
function WD = fcn(x,Ts,P)
    % Estados atuais
    WTD=x(1);  WQA=x(2);
    WRC=x(3);  WAP=x(4);
    WD=x(5);

    % Extrai constantes dos parâmetros
    Ktd=P(1);     Kqa=P(2);      Krc=P(3);      Kap=P(4);
    Ptd=P(5);     Pqa=P(6);      Prc=P(7);      Pap=P(8);
    AlfaQA=P(9);  AlfaRC=P(10);  AlfaAP=P(11);

    % Entrada é a vazão de saida do tanque WAP, descontados os retrabalhos de AP
    Qin=(1-AlfaAP)*Kap*sqrt(WAP+Pap);  

    % Expressão da Eq.Diferencial
    Derivada = Qin;    % Só acumula infinitamente o trabalho realizado
    
    % Atualização do Estado
    WD = WD + Ts*Derivada;

    % Proteção, já que não faz sentido quantidades negativas para reciclos
    WD=max(WD,0);
end

== matlab function Modelos/Task 05/MATLAB Function ==
  data: enable input; Done output; Work input
function Done = fcn(enable,Work)
  
  if (enable) & (sum(Work(1:4))==0)   % Habilitado mas não tem mais nada para fazer
    Done = 1;  % Trabalho feito
  else
    Done = 0;  % Ainda há trabalho por fazer
  end
end
